simulink model "AFC_ensemble_other"  (R2022a)
settings: Solver=ode15s  StartTime=0.0  StopTime=T  MaxStep=.01  RelTol=1e-3
InitFcn:
  | seed_PA = randi(20000);
  | seed_ES = randi(20000);
StartFcn:
  | seed_PA = randi(20000);
  | seed_ES = randi(20000);
undefined symbols (not defined in the file): actionTable, actionUB, AF_ref_normal, AF_ref_power, AF_sensor_tol, change_freq_ES, change_freq_PA, edge_mu_max, fault_time, fuel_inj_max, fuel_inj_min, fuel_inj_tol, isAvg, isPred, isTerminate, isVote, kappa_tol, MAF_sensor_tol, max_Engine_Speed, max_Pedal_Angle, min_Engine_Speed, min_Pedal_Angle, mu_tol_normal, power_threshold, pump_tol, rewardToIndex, rewardUB1, rewardUB2, rewardWeights, stateTable, steady_mu_max, tau_ww_tol, time_tol, tranTable
libraries: rllib x9, simulink x2, dspstat3 x1
Description:
  | Modeling Engine Timing Using Triggered Subsystems
  | 
  | This example presents a model of a four-cylinder spark ignition engine
  | and demonstrates Simulink(R) capabilities to model an internal combustion
  | engine from the throttle to the crankshaft output. We used well-defined
  | physical principles supplemented, where appropriate, with empirical
  | relationships that describe the systems dynamic behavior without
  | introducing unnecessary complexity.
settings Model: ExtModeTrigMode=oneshot  ExtModeArmWhenConnect=off  Creator=The MathWorks Inc.  LastModifiedBy=momentumlab
settings SolverCC: ZeroCrossControl=DisableAll  AlgebraicLoopSolver=TrustRegion
settings DataIOCC: ExternalInput=[t__, u__]  SaveFormat=StructureWithTime  DSMLogging=off  ReturnWorkspaceOutputs=off
settings OptimizationCC: BlockReduction=off  BooleanDataType=off  LifeSpan=inf
settings DebuggingCC: SaveWithParameterizedLinksMsg=none  UnderspecifiedInitializationDetection=Classic  MergeDetectMultiDrivingBlocksExec=none  SignalResolutionControl=TryResolveAllWithWarning  ParameterPrecisionLossMsg=none  UnconnectedInputMsg=warning  UnconnectedOutputMsg=warning  UnconnectedLineMsg=warning  SFUnexpectedBacktrackingDiag=warning  SFNoUnconditionalDefaultTransitionDiag=warning  SFExecutionAtInitializationDiag=none  SFMachineParentedDataDiag=warning  ArithmeticOperatorsInVariantConditions=warning
settings HardwareCC: ProdBitPerPointer=32  ProdBitPerSizeT=32  ProdBitPerPtrDiffT=32  ProdLargestAtomicFloat=None  ProdIntDivRoundTo=Undefined  ProdEndianess=Unspecified  ProdWordSize=32  ProdHWDeviceType=32-bit Generic  TargetBitPerLong=64  TargetBitPerPointer=64  TargetBitPerSizeT=64  TargetBitPerPtrDiffT=64  TargetLongLongMode=on  TargetIntDivRoundTo=Zero  TargetEndianess=LittleEndian  TargetWordSize=64  TargetHWDeviceType=MATLAB Host  ProdEqTarget=off
settings ModelReferenceCC: PropagateSignalLabelsOutOfModel=off
settings SFSimCC: SimUseLocalCustomCode=off  CustomCodeUndefinedFunction=UseInterfaceOnly
settings RTWCC: RTWUseLocalCustomCode=off  DLArmComputeVersion=19.05
settings CodeAppCC: StateflowObjectComments=on
settings GRTTargetCC: TargetLangStandard=C89/C90 (ANSI)
settings ConfigComp: CovMetricSettings=d  CovSaveCumulativeToWorkspaceVar=on  CovSaveSingleToWorkspaceVar=on  CovExternalEMLEnable=off

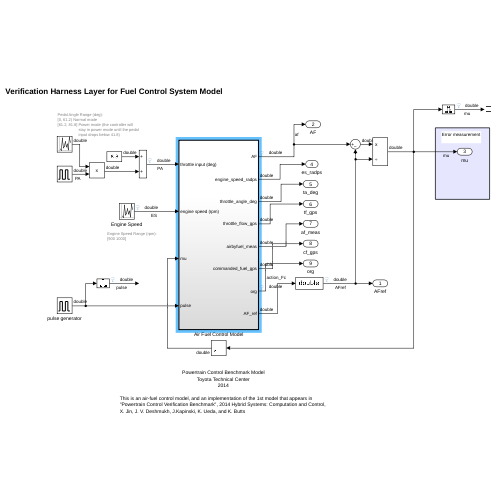
[thumbnail: Simulink's stored preview of the top-level diagram]
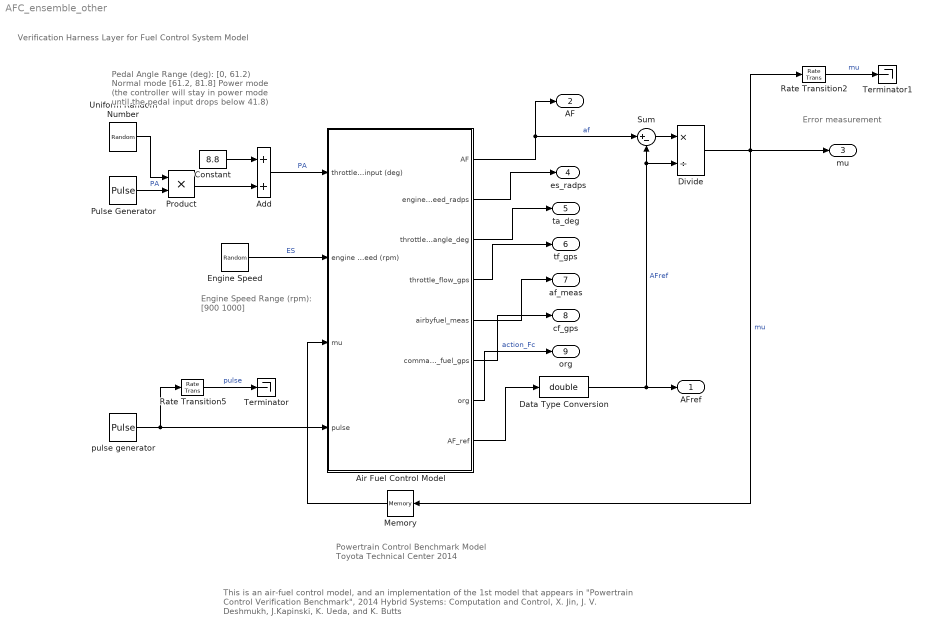
== system AFC_ensemble_other ==
  note: Error measurement
  note: Pedal Angle Range (deg):
      | [0, 61.2) Normal mode
      | [61.2, 81.8] Power mode (the controller will
      |                    stay in power mode until the pedal
      |                    input drops below 41.8)
  note: This is an air-fuel control model, and an implementation of the 1st model that appears in
      | "Powertrain Control Verification Benchmark", 2014 Hybrid Systems: Computation and Control,
      | X. Jin, J. V. Deshmukh, J.Kapinski, K. Ueda, and K. Butts
  note: Engine Speed Range (rpm):
      | [900 1000]
  note: Powertrain Control Benchmark Model
      | Toyota Technical Center
      | 2014
  note: Verification Harness Layer for Fuel Control System Model
  Add : Sum
  Air Fuel Control Model : Subsystem  Priority=1  TreatAsAtomicUnit=on
  Constant : Constant  Value=8.8
  Data Type Conversion : DataTypeConversion  OutDataTypeStr=double  SaturateOnIntegerOverflow=off  RndMeth=Floor
  Divide : Product  Inputs=*/
  Engine Speed : UniformRandomNumber  Minimum=min_Engine_Speed  Maximum=max_Engine_Speed  Seed=seed_ES  SampleTime=change_freq_ES  VectorParams1D=off
  Memory : Memory
  Product : Product
  Pulse Generator : DiscretePulseGenerator  PulseType=Time based  Period=change_freq_PA  PulseWidth=50
  Rate Transition2 : RateTransition  OutPortSampleTime=Ts_sample
  Rate Transition5 : RateTransition  OutPortSampleTime=Ts_sample
  Sum : Sum  Inputs=|+-
  Terminator : Terminator
  Terminator1 : Terminator
  Uniform Random Number : UniformRandomNumber  Minimum=min_Pedal_Angle  Maximum=max_Pedal_Angle  Seed=seed_PA  SampleTime=change_freq_PA
  pulse generator : DiscretePulseGenerator  PulseType=Time based  Period=change_freq_ES  PulseWidth=50  PhaseDelay=0.3
  AFref : Outport  VectorParamsAs1DForOutWhenUnconnected=off
  AF : Outport  Port=2  VectorParamsAs1DForOutWhenUnconnected=off
  mu : Outport  Port=3  VectorParamsAs1DForOutWhenUnconnected=off
  es_radps : Outport  Port=4
  ta_deg : Outport  Port=5
  tf_gps : Outport  Port=6
  af_meas : Outport  Port=7
  cf_gps : Outport  Port=8
  org : Outport  Port=9
  wires:
  Air Fuel Control Model/1(AF) -> AF/1, Sum/1  "af"
  Add/1 -> Air Fuel Control Model/1(throttle input (deg))  "PA"
  Air Fuel Control Model/8(AF_ref) -> Data Type Conversion/1
  Engine Speed/1 -> Air Fuel Control Model/2(engine speed (rpm))  "ES"
  Data Type Conversion/1 -> Sum/2, Divide/2, AFref/1  "AFref"
  Sum/1 -> Divide/1
  Air Fuel Control Model/2(engine_speed_radps) -> es_radps/1
  Air Fuel Control Model/3(throttle_angle_deg) -> ta_deg/1
  Air Fuel Control Model/4(throttle_flow_gps) -> tf_gps/1
  Air Fuel Control Model/5(airbyfuel_meas) -> af_meas/1
  Air Fuel Control Model/6(commanded_fuel_gps) -> cf_gps/1
  Air Fuel Control Model/7(org) -> org/1  "action_Fc"
  Divide/1 -> mu/1, Memory/1, Rate Transition2/1  "mu"
  Memory/1 -> Air Fuel Control Model/3(mu)
  Pulse Generator/1 -> Product/2  "PA"
  Uniform Random Number/1 -> Product/1
  Constant/1 -> Add/1
  Product/1 -> Add/2
  pulse generator/1 -> Rate Transition5/1, Air Fuel Control Model/4(pulse)
  Rate Transition5/1 -> Terminator/1  "pulse"
  Rate Transition2/1 -> Terminator1/1  "mu"

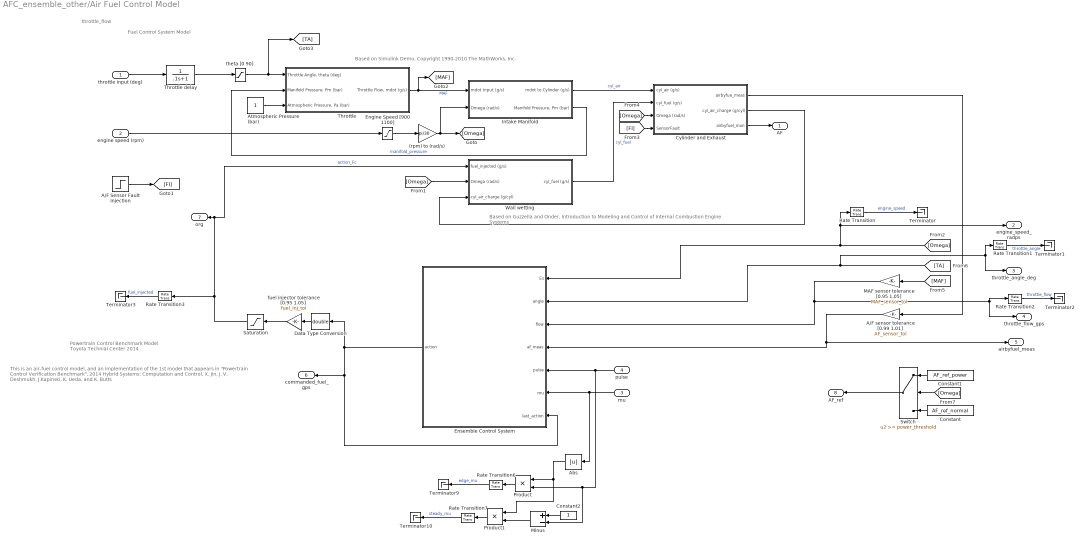
== system AFC_ensemble_other/Air Fuel Control Model ==
  note: throttle_flow
  note: Based on Simulink Demo, Copyright 1990-2010 The MathWorks, Inc.
  note: Based on Guzzella and Onder, Introduction to Modeling and Control of Internal Combustion Engine Systems
  note: Fuel Control System Model
  note: This is an air-fuel control model, and an implementation of the 1st model that appears in
      | "Powertrain Control Verification Benchmark", 2014 Hybrid Systems: Computation and Control,
      | X. Jin, J. V. Deshmukh, J.Kapinski, K. Ueda, and K. Butts
  note: Powertrain Control Benchmark Model
      | Toyota Technial Center
      | 2014
  throttle input (deg) : Inport  Description=[0, 81.2]
      settings: AttributesFormatString=%<Description>
  engine speed (rpm) : Inport  Description=[900,1100]  Port=2
      settings: AttributesFormatString=%<Description>
  mu : Inport  Port=3
  pulse : Inport  Port=4
  (rpm) to (rad/s) : Gain  Gain=pi/30
  A/F Sensor Fault Injection : Step  Time=fault_time  SampleTime=0
      settings: AttributesFormatString=1: Failure\n0: Normal
  A/F sensor tolerance [0.99 1.01] : Gain  Gain=AF_sensor_tol
  Abs : Abs  SaturateOnIntegerOverflow=off
  Atmospheric Pressure (bar) : Constant
  Constant : Constant  Value=AF_ref_normal
  Constant1 : Constant  Value=AF_ref_power
  Constant2 : Constant
  Cylinder and Exhaust : Subsystem
  Data Type Conversion : DataTypeConversion  OutDataTypeStr=double  SaturateOnIntegerOverflow=off  RndMeth=Floor
  Engine Speed [900 1100] : Saturate  UpperLimit=1100  LowerLimit=900
  Ensemble Control System : Subsystem
  Intake Manifold : Subsystem
  MAF sensor tolerance [0.95 1.05] : Gain  Gain=MAF_sensor_tol
  Minus : Sum  Inputs=+-
  Product : Product
  Product1 : Product
  Rate Transition{,1..3,6..7} (6 alike) : RateTransition  OutPortSampleTime=Ts_sample
  Saturation : Saturate  UpperLimit=fuel_inj_max  LowerLimit=fuel_inj_min
  Switch : Switch  Threshold=power_threshold  SaturateOnIntegerOverflow=off  InputSameDT=off
  Terminator{,1..3,9..10} (6 alike) : Terminator
  Throttle : Subsystem
  Throttle delay : TransferFcn  Denominator=[.1 1]
  Wall wetting : Subsystem
  fuel injector tolerance [0.95 1.05] : Gain  Gain=fuel_inj_tol
  theta [0 90] : Saturate  UpperLimit=90  LowerLimit=0
  AF : Outport  VectorParamsAs1DForOutWhenUnconnected=off
  engine_speed_radps : Outport  Port=2
  throttle_angle_deg : Outport  Port=3
  throttle_flow_gps : Outport  Port=4
  airbyfuel_meas : Outport  Port=5
  commanded_fuel_gps : Outport  Port=6
  org : Outport  Port=7
  AF_ref : Outport  Port=8
  wires:
  (rpm) to (rad/s)/1 -> [Omega], Intake Manifold/2(Omega (rad/s))
  Data Type Conversion/1 -> fuel injector tolerance [0.95 1.05]/1
  theta [0 90]/1 -> Throttle/1("Throttle Angle, theta (deg)"), [TA]
  Engine Speed [900 1100]/1 -> (rpm) to (rad/s)/1
  Cylinder and Exhaust/3("airbyfuel_mon ") -> AF/1
  MAF sensor tolerance [0.95 1.05]/1 -> Ensemble Control System/3(flow), throttle_flow_gps/1, Rate Transition2/1
  A/F sensor tolerance [0.99 1.01]/1 -> airbyfuel_meas/1, Ensemble Control System/4(af_meas)
  [MAF] -> MAF sensor tolerance [0.95 1.05]/1
  Cylinder and Exhaust/1(airbyfue_meas) -> A/F sensor tolerance [0.99 1.01]/1
  Throttle/1("Throttle Flow, mdot (g/s)") -> [MAF], Intake Manifold/1(mdot Input (g/s))  "MAF"
  Intake Manifold/2("Manifold Pressure, Pm (bar)") -> Throttle/2("Manifold Pressure, Pm (bar)")  "manifold_pressure"
  Atmospheric Pressure (bar)/1 -> Throttle/3("Atmospheric Pressure, Pa (bar) ")
  Wall wetting/1(cyl_fuel (g/s)) -> Cylinder and Exhaust/2(cyl_fuel (g/s))  "cyl_fuel"
  Intake Manifold/1(mdot to Cylinder (g/s)) -> Cylinder and Exhaust/1(cyl_air (g/s))  "cyl_air"
  [Omega] -> Cylinder and Exhaust/3(Omega (rad/s))
  [Omega] -> Wall wetting/2(Omega (rad/s))
  Cylinder and Exhaust/2(cyl_air_charge (g/cyl)) -> Wall wetting/3(cyl_air_charge (g/cyl))
  A/F Sensor Fault Injection/1 -> [FI]
  [FI] -> Cylinder and Exhaust/4(SensorFault)
  [TA] -> Ensemble Control System/2(angle), Rate Transition1/1, throttle_angle_deg/1
  throttle input (deg)/1 -> Throttle delay/1
  engine speed (rpm)/1 -> Engine Speed [900 1100]/1
  Throttle delay/1 -> theta [0 90]/1
  fuel injector tolerance [0.95 1.05]/1 -> Saturation/1
  Saturation/1 -> Rate Transition3/1, Wall wetting/1(fuel_injected (g/s)), org/1  "action_Fc"
  [Omega] -> Switch/2
  Constant1/1 -> Switch/1
  Constant/1 -> Switch/3
  Switch/1 -> AF_ref/1
  Rate Transition/1 -> Terminator/1  "engine_speed"
  [Omega] -> Ensemble Control System/1(Es), engine_speed_radps/1, Rate Transition/1
  Rate Transition1/1 -> Terminator1/1  "throttle_angle"
  Rate Transition2/1 -> Terminator2/1  "throttle_flow"
  Rate Transition3/1 -> Terminator3/1  "fuel_injected"
  Ensemble Control System/1(action) -> Data Type Conversion/1, Ensemble Control System/7(last_action), commanded_fuel_gps/1
  Rate Transition6/1 -> Terminator9/1  "edge_mu"
  Abs/1 -> Product1/1, Product/1
  Constant2/1 -> Minus/1
  pulse/1 -> Product/2, Minus/2, Ensemble Control System/5(pulse)
  Product1/1 -> Rate Transition7/1
  Product/1 -> Rate Transition6/1
  Rate Transition7/1 -> Terminator10/1  "steady_mu"
  mu/1 -> Abs/1, Ensemble Control System/6(mu)
  Minus/1 -> Product1/2

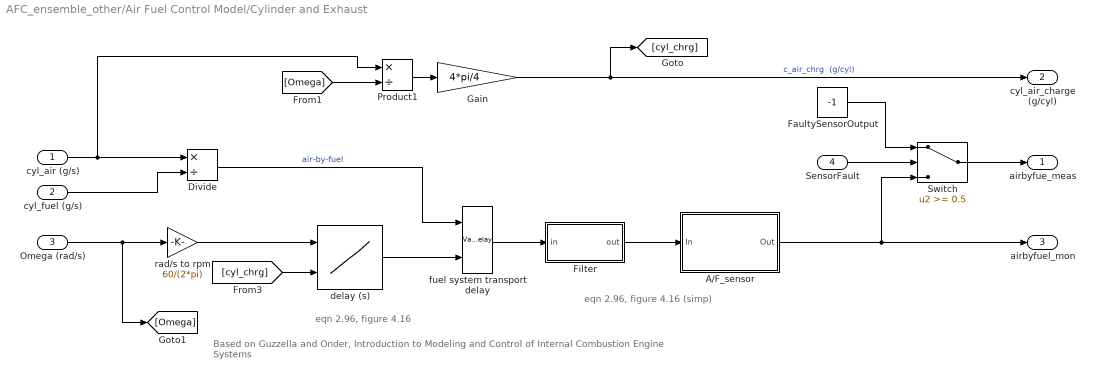
== system AFC_ensemble_other/Air Fuel Control Model/Cylinder and Exhaust ==
  note: Based on Guzzella and Onder, Introduction to Modeling and Control of Internal Combustion Engine Systems
  note: eqn 2.96, figure 4.16
  note: eqn 2.96, figure 4.16 (simp)
  cyl_air (g/s) : Inport
  cyl_fuel (g/s) : Inport  Port=2
  Omega (rad/s) : Inport  Port=3
  SensorFault : Inport  Port=4
  A/F_sensor : Subsystem
  Divide : Product  Inputs=*/
  FaultySensorOutput : Constant  Value=-1
  Filter : Subsystem
  Gain : Gain  Gain=4*pi/4
  Product1 : Product  Inputs=*/  RndMeth=Zero
  Switch : Switch  Threshold=0.5  SaturateOnIntegerOverflow=off  InputSameDT=off
  delay (s) : Lookup_n-D  BreakpointsForDimension1=[800,1000,1500,2000,3000]  BreakpointsForDimension2=[0.05,0.15,0.2,0.25]  Table=reshape([0.8,0.6,0.4,0.3,0.2,0.4,0.3,0.2,0.2,0.2,0.3,0.25,0.2,0.2,0.2,0.25,0.2,0.2,0.2,0.2],5,4)  UseLastTableValue=on  RndMeth=Simplest
      settings: InputPortMap=u0,u1
  fuel system transport delay : VariableTransportDelay  VariableDelayType=Variable transport delay  MaximumDelay=10  InitialOutput=14.7  MaximumPoints=20480
  rad/s to rpm : Gain  Gain=60/(2*pi)
  airbyfue_meas : Outport  VectorParamsAs1DForOutWhenUnconnected=off
  cyl_air_charge (g/cyl) : Outport  Port=2  VectorParamsAs1DForOutWhenUnconnected=off
  "airbyfuel_mon " : Outport  Port=3  VectorParamsAs1DForOutWhenUnconnected=off
  wires:
  cyl_air (g/s)/1 -> Divide/1, Product1/1
  [Omega] -> Product1/2
  Product1/1 -> Gain/1
  Gain/1 -> [cyl_chrg], cyl_air_charge (g/cyl)/1  "c_air_chrg  (g/cyl)"
  [cyl_chrg] -> delay (s)/2
  cyl_fuel (g/s)/1 -> Divide/2
  Omega (rad/s)/1 -> [Omega], rad/s to rpm/1
  rad/s to rpm/1 -> delay (s)/1
  delay (s)/1 -> fuel system transport delay/2
  fuel system transport delay/1 -> Filter/1(in)
  Switch/1 -> airbyfue_meas/1
  Divide/1 -> fuel system transport delay/1  "air-by-fuel"
  Filter/1(out) -> A/F_sensor/1(In)
  FaultySensorOutput/1 -> Switch/1
  SensorFault/1 -> Switch/2
  A/F_sensor/1(Out) -> Switch/3, "airbyfuel_mon "/1

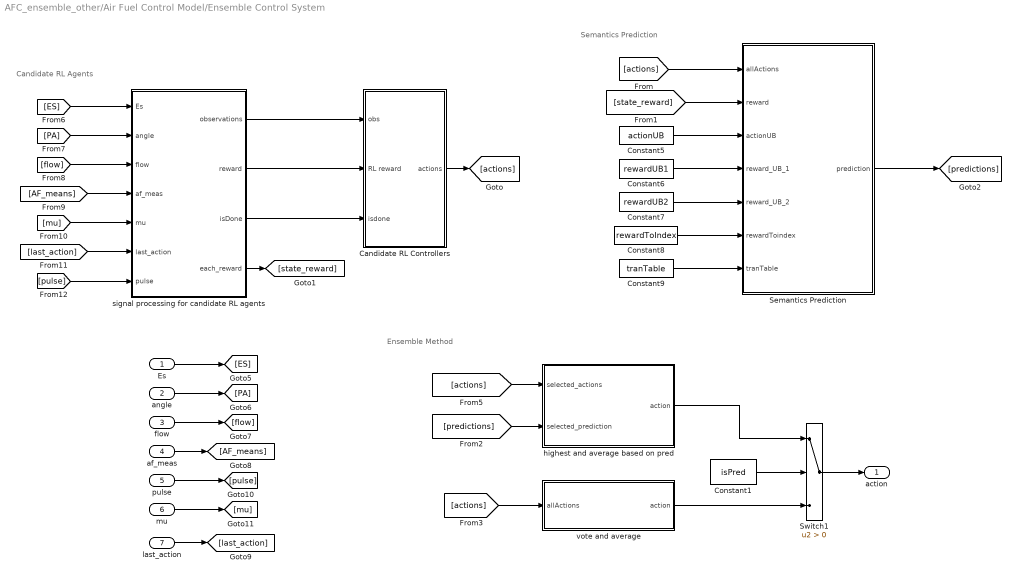
== system AFC_ensemble_other/Air Fuel Control Model/Ensemble Control System ==
  note: Candidate RL Agents
  note: Semantics Prediction
  note: Ensemble Method
  Es : Inport
  angle : Inport  Port=2
  flow : Inport  Port=3
  af_meas : Inport  Port=4
  pulse : Inport  Port=5
  mu : Inport  Port=6
  last_action : Inport  Port=7
  Candidate RL Controllers : Subsystem
  Constant1 : Constant  Value=isPred
  Constant5 : Constant  Value=actionUB
  Constant6 : Constant  Value=rewardUB1
  Constant7 : Constant  Value=rewardUB2
  Constant8 : Constant  Value=rewardToIndex
  Constant9 : Constant  Value=tranTable
  Semantics Prediction : Subsystem
  Switch1 : Switch  Criteria=u2 > Threshold  SaturateOnIntegerOverflow=off  InputSameDT=off
  highest and average based on pred : Subsystem
  signal processing for candidate RL agents : Subsystem
  vote and average : Subsystem
  action : Outport
  wires:
  last_action/1 -> [last_action]
  signal processing for candidate RL agents/3(isDone) -> Candidate RL Controllers/3(isdone)
  Constant8/1 -> Semantics Prediction/6(rewardToindex)
  Candidate RL Controllers/1(actions) -> [actions]
  Semantics Prediction/1(prediction) -> [predictions]
  signal processing for candidate RL agents/4(each_reward) -> [state_reward]
  [state_reward] -> Semantics Prediction/2(reward)
  Constant9/1 -> Semantics Prediction/7(tranTable)
  Constant5/1 -> Semantics Prediction/3(actionUB)
  Constant6/1 -> Semantics Prediction/4(reward_UB_1)
  [actions] -> Semantics Prediction/1(allActions)
  Constant7/1 -> Semantics Prediction/5(reward_UB_2)
  signal processing for candidate RL agents/2(reward) -> Candidate RL Controllers/2(RL reward)
  signal processing for candidate RL agents/1(observations) -> Candidate RL Controllers/1(obs)
  Es/1 -> [ES]
  angle/1 -> [PA]
  flow/1 -> [flow]
  af_meas/1 -> [AF_means]
  pulse/1 -> [pulse]
  mu/1 -> [mu]
  [ES] -> signal processing for candidate RL agents/1(Es)
  [PA] -> signal processing for candidate RL agents/2(angle)
  [flow] -> signal processing for candidate RL agents/3(flow)
  [AF_means] -> signal processing for candidate RL agents/4(af_meas)
  [mu] -> signal processing for candidate RL agents/5(mu)
  [last_action] -> signal processing for candidate RL agents/6(last_action)
  [pulse] -> signal processing for candidate RL agents/7(pulse)
  Constant1/1 -> Switch1/2
  [actions] -> vote and average/1(allActions)
  vote and average/1(action) -> Switch1/3
  highest and average based on pred/1(action) -> Switch1/1
  Switch1/1 -> action/1
  [predictions] -> highest and average based on pred/2(selected_prediction)
  [actions] -> highest and average based on pred/1(selected_actions)

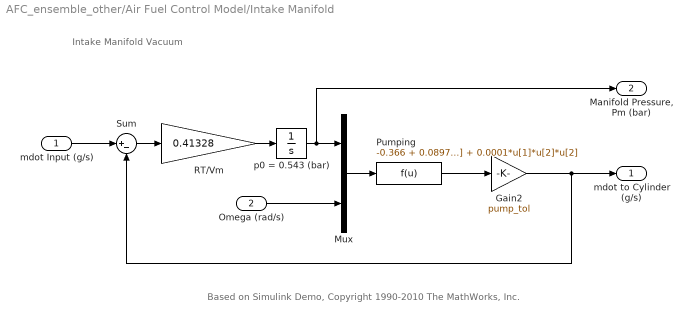
== system AFC_ensemble_other/Air Fuel Control Model/Intake Manifold ==
  note: Intake Manifold Vacuum
  note: Based on Simulink Demo, Copyright 1990-2010 The MathWorks, Inc.
  mdot Input (g/s) : Inport
  Omega (rad/s) : Inport  Port=2
  Gain2 : Gain  Gain=pump_tol  ParamDataTypeStr=single  OutDataTypeStr=Inherit: Inherit via back propagation  RndMeth=Simplest  SaturateOnIntegerOverflow=on
      settings: AttributesFormatString=pumping tolerance [0.9 1.1]
  Mux : Mux  Inputs=2
  Pumping : Fcn  Expr=-0.366 + 0.08979*u[1]*u[2] - 0.0337*u[2]*u[1]*u[1] + 0.0001*u[1]*u[2]*u[2]
  RT/Vm : Gain  Gain=0.41328  SaturateOnIntegerOverflow=on  OutDataTypeStr=Inherit: Same as input  ParamDataTypeStr=Inherit: Same as input
  Sum : Sum  Inputs=|+-  InputSameDT=on  SaturateOnIntegerOverflow=on  OutDataTypeStr=Inherit: Same as first input
  p0 = 0.543 (bar) : Integrator  InitialCondition=0.982
  mdot to Cylinder (g/s) : Outport  InitialOutput=0  VectorParamsAs1DForOutWhenUnconnected=off
  "Manifold Pressure, Pm (bar)" : Outport  Port=2  InitialOutput=0  VectorParamsAs1DForOutWhenUnconnected=off
  wires:
  mdot Input (g/s)/1 -> Sum/1
  RT/Vm/1 -> p0 = 0.543 (bar)/1
  Omega (rad/s)/1 -> Mux/2
  Mux/1 -> Pumping/1
  p0 = 0.543 (bar)/1 -> Mux/1, "Manifold Pressure, Pm (bar)"/1
  Sum/1 -> RT/Vm/1
  Pumping/1 -> Gain2/1
  Gain2/1 -> Sum/2, mdot to Cylinder (g/s)/1

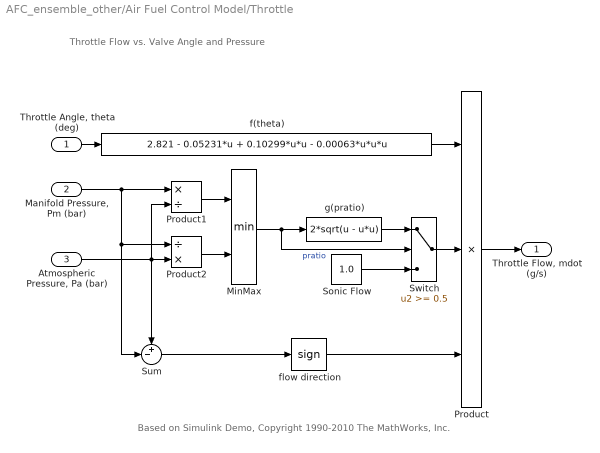
== system AFC_ensemble_other/Air Fuel Control Model/Throttle ==
  note: Throttle Flow vs. Valve Angle and Pressure
  note: Based on Simulink Demo, Copyright 1990-2010 The MathWorks, Inc.
  "Throttle Angle, theta (deg)" : Inport
  "Manifold Pressure, Pm (bar)" : Inport  Port=2
  "Atmospheric Pressure, Pa (bar) " : Inport  Port=3
  MinMax : MinMax  Inputs=2  InputSameDT=on  SaturateOnIntegerOverflow=on
  Product : Product  Inputs=3  InputSameDT=on  RndMeth=Zero  SaturateOnIntegerOverflow=on  OutDataTypeStr=Inherit: Same as first input
  Product1 : Product  Inputs=*/  InputSameDT=on  RndMeth=Zero  SaturateOnIntegerOverflow=on  OutDataTypeStr=Inherit: Same as first input
  Product2 : Product  Inputs=/*  InputSameDT=on  RndMeth=Zero  SaturateOnIntegerOverflow=on  OutDataTypeStr=Inherit: Same as first input
  "Sonic Flow " : Constant  Value=1.0
  Sum : Sum  Inputs=+-|  InputSameDT=on  SaturateOnIntegerOverflow=on  OutDataTypeStr=Inherit: Same as first input
  Switch : Switch  Threshold=0.5
  f(theta) : Fcn  Expr=2.821 - 0.05231*u + 0.10299*u*u - 0.00063*u*u*u
  flow direction : Signum
  g(pratio) : Fcn  Expr=2*sqrt(u - u*u)
  "Throttle Flow, mdot (g/s)" : Outport  InitialOutput=0  VectorParamsAs1DForOutWhenUnconnected=off
  wires:
  "Manifold Pressure, Pm (bar)"/1 -> Sum/2, Product2/1, Product1/1
  Product2/1 -> MinMax/2
  Product1/1 -> MinMax/1
  "Atmospheric Pressure, Pa (bar) "/1 -> Sum/1, Product2/2, Product1/2
  g(pratio)/1 -> Switch/1
  "Sonic Flow "/1 -> Switch/3
  Switch/1 -> Product/2
  flow direction/1 -> Product/3
  Sum/1 -> flow direction/1
  MinMax/1 -> g(pratio)/1, Switch/2  "pratio"
  "Throttle Angle, theta (deg)"/1 -> f(theta)/1
  Product/1 -> "Throttle Flow, mdot (g/s)"/1
  f(theta)/1 -> Product/1

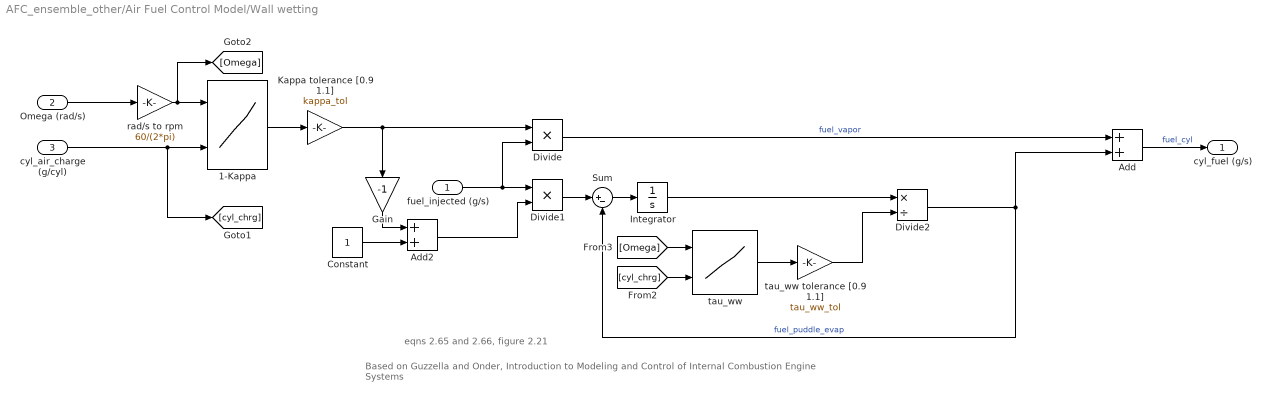
== system AFC_ensemble_other/Air Fuel Control Model/Wall wetting ==
  note: Based on Guzzella and Onder, Introduction to Modeling and Control of Internal Combustion Engine Systems
  note: eqns 2.65 and 2.66, figure 2.21
  fuel_injected (g/s) : Inport
  Omega (rad/s) : Inport  Port=2
  cyl_air_charge (g/cyl) : Inport  Port=3
  1-Kappa : Lookup_n-D  BreakpointsForDimension1=[1000,1500,2000,2500,3000]  BreakpointsForDimension2=[.1,.2,.3,.4]  Table=reshape([0.8,.7,.7,.8,.9,.7,.66,.65,.73,.85,.66,.66,.63,.66,.8,.6,.6,.6,.6,.7],5,4)  UseLastTableValue=on  RndMeth=Simplest
      settings: InputPortMap=u0,u1
  Add : Sum
  Add2 : Sum
  Constant : Constant
  Divide : Product  Inputs=**
  Divide1 : Product  Inputs=**
  Divide2 : Product  Inputs=*/
  Gain : Gain  Gain=-1
  Integrator : Integrator  InitialCondition=.0112
  Kappa tolerance [0.9 1.1] : Gain  Gain=kappa_tol
  Sum : Sum  Inputs=|+-
  rad/s to rpm : Gain  Gain=60/(2*pi)
  tau_ww : Lookup_n-D  BreakpointsForDimension1=[1000,1500,2000,2500,3000]  BreakpointsForDimension2=[0.1,0.2,0.3,0.4]  Table=reshape([.4,.3,.35,.3,.2,.22,.22,.4,.35,.5,.20,.22,.5,.4,.35,.35,.3,.45,.5,.4],5,4)  UseLastTableValue=on  RndMeth=Simplest
      settings: InputPortMap=u0,u1
  tau_ww tolerance [0.9 1.1] : Gain  Gain=tau_ww_tol
  cyl_fuel (g/s) : Outport  VectorParamsAs1DForOutWhenUnconnected=off
  wires:
  1-Kappa/1 -> Kappa tolerance [0.9 1.1]/1
  fuel_injected (g/s)/1 -> Divide/2, Divide1/1
  Divide/1 -> Add/1  "fuel_vapor"
  Add/1 -> cyl_fuel (g/s)/1  "fuel_cyl"
  Integrator/1 -> Divide2/1
  Divide1/1 -> Sum/1
  Sum/1 -> Integrator/1
  Divide2/1 -> Add/2, Sum/2  "fuel_puddle_evap"
  Add2/1 -> Divide1/2
  cyl_air_charge (g/cyl)/1 -> 1-Kappa/2, [cyl_chrg]
  [cyl_chrg] -> tau_ww/2
  tau_ww/1 -> tau_ww tolerance [0.9 1.1]/1
  Gain/1 -> Add2/1
  Constant/1 -> Add2/2
  rad/s to rpm/1 -> [Omega], 1-Kappa/1
  Omega (rad/s)/1 -> rad/s to rpm/1
  Kappa tolerance [0.9 1.1]/1 -> Divide/1, Gain/1
  tau_ww tolerance [0.9 1.1]/1 -> Divide2/2
  [Omega] -> tau_ww/1

== system AFC_ensemble_other/Air Fuel Control Model/Cylinder and Exhaust/A//F_sensor ==
  In : Inport
  A/F_sensor : Gain  OutDataTypeStr=double
  Filter : Subsystem
  Out : Outport  VectorParamsAs1DForOutWhenUnconnected=off
  wires:
  A/F_sensor/1 -> Out/1
  In/1 -> Filter/1(In)
  Filter/1(Out) -> A/F_sensor/1

== system AFC_ensemble_other/Air Fuel Control Model/Cylinder and Exhaust/Filter ==
  in : Inport
  Gain1 : Gain  Gain=10
  Integrator : Integrator  InitialCondition=14.7
  Sum : Sum  Inputs=|+-
  out : Outport  VectorParamsAs1DForOutWhenUnconnected=off
  wires:
  Integrator/1 -> out/1, Sum/2
  in/1 -> Sum/1
  Gain1/1 -> Integrator/1
  Sum/1 -> Gain1/1

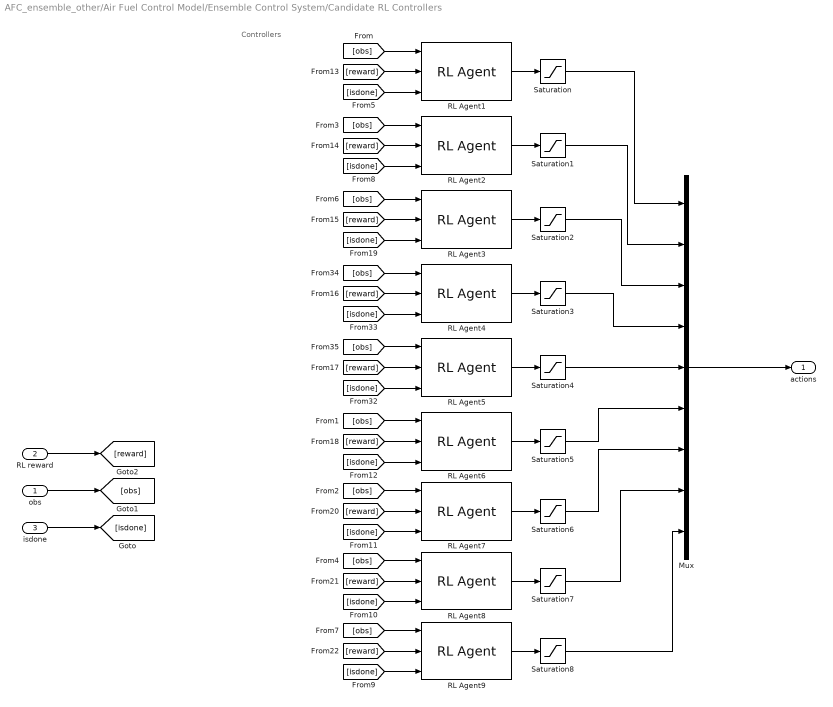
== system AFC_ensemble_other/Air Fuel Control Model/Ensemble Control System/Candidate RL Controllers ==
  note: Controllers
  obs : Inport
  RL reward : Inport  Port=2
  isdone : Inport  Port=3
  Mux : Mux  Inputs=9
  RL Agent1 : rllib/RL Agent  Agent=agent1  ExternalActionAsInput=off  ProvideLastAction=off  ProvideCumRwd=off  TreatAsDirectFeedthrough=on  UseStrictObservationDataTypes=off
  RL Agent2 : rllib/RL Agent  Agent=agent2  ExternalActionAsInput=off  ProvideLastAction=off  ProvideCumRwd=off  TreatAsDirectFeedthrough=on  UseStrictObservationDataTypes=off
  RL Agent3 : rllib/RL Agent  Agent=agent3  ExternalActionAsInput=off  ProvideLastAction=off  ProvideCumRwd=off  TreatAsDirectFeedthrough=on  UseStrictObservationDataTypes=off
  RL Agent4 : rllib/RL Agent  Agent=agent3  ExternalActionAsInput=off  ProvideLastAction=off  ProvideCumRwd=off  TreatAsDirectFeedthrough=on  UseStrictObservationDataTypes=off
  RL Agent5 : rllib/RL Agent  Agent=agent3  ExternalActionAsInput=off  ProvideLastAction=off  ProvideCumRwd=off  TreatAsDirectFeedthrough=on  UseStrictObservationDataTypes=off
  RL Agent6 : rllib/RL Agent  Agent=agent6  ExternalActionAsInput=off  ProvideLastAction=off  ProvideCumRwd=off  TreatAsDirectFeedthrough=on  UseStrictObservationDataTypes=off
  RL Agent7 : rllib/RL Agent  Agent=agent7  ExternalActionAsInput=off  ProvideLastAction=off  ProvideCumRwd=off  TreatAsDirectFeedthrough=on  UseStrictObservationDataTypes=off
  RL Agent8 : rllib/RL Agent  Agent=agent8  ExternalActionAsInput=off  ProvideLastAction=off  ProvideCumRwd=off  TreatAsDirectFeedthrough=on  UseStrictObservationDataTypes=off
  RL Agent9 : rllib/RL Agent  Agent=agent9  ExternalActionAsInput=off  ProvideLastAction=off  ProvideCumRwd=off  TreatAsDirectFeedthrough=on  UseStrictObservationDataTypes=off
  Saturation{,1..8} (9 alike) : Saturate  UpperLimit=fuel_inj_max  LowerLimit=fuel_inj_min
  actions : Outport
  wires:
  [obs] -> RL Agent7/1
  [obs] -> RL Agent4/1
  [obs] -> RL Agent3/1
  Saturation3/1 -> Mux/4
  [obs] -> RL Agent1/1
  [isdone] -> RL Agent1/3
  [obs] -> RL Agent2/1
  [obs] -> RL Agent5/1
  RL Agent1/1 -> Saturation/1
  [isdone] -> RL Agent8/3
  [isdone] -> RL Agent6/3
  Saturation/1 -> Mux/1
  RL Agent6/1 -> Saturation5/1
  Saturation4/1 -> Mux/5
  RL Agent3/1 -> Saturation2/1
  [isdone] -> RL Agent2/3
  [isdone] -> RL Agent7/3
  RL Agent8/1 -> Saturation7/1
  Saturation1/1 -> Mux/2
  [isdone] -> RL Agent5/3
  Mux/1 -> actions/1
  [obs] -> RL Agent6/1
  [isdone] -> RL Agent3/3
  RL Agent5/1 -> Saturation4/1
  RL Agent4/1 -> Saturation3/1
  RL Agent7/1 -> Saturation6/1
  RL Agent2/1 -> Saturation1/1
  [obs] -> RL Agent8/1
  Saturation2/1 -> Mux/3
  [isdone] -> RL Agent4/3
  RL Agent9/1 -> Saturation8/1
  [obs] -> RL Agent9/1
  [isdone] -> RL Agent9/3
  Saturation5/1 -> Mux/6
  Saturation6/1 -> Mux/7
  Saturation7/1 -> Mux/8
  Saturation8/1 -> Mux/9
  isdone/1 -> [isdone]
  obs/1 -> [obs]
  RL reward/1 -> [reward]
  [reward] -> RL Agent1/2
  [reward] -> RL Agent2/2
  [reward] -> RL Agent3/2
  [reward] -> RL Agent4/2
  [reward] -> RL Agent5/2
  [reward] -> RL Agent6/2
  [reward] -> RL Agent7/2
  [reward] -> RL Agent8/2
  [reward] -> RL Agent9/2

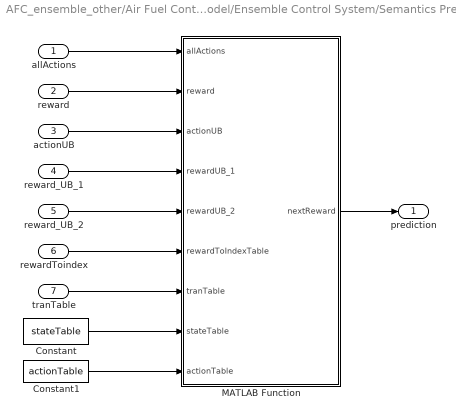
== system AFC_ensemble_other/Air Fuel Control Model/Ensemble Control System/Semantics Prediction ==
  allActions : Inport
  reward : Inport  Port=2
  actionUB : Inport  Port=3
  reward_UB_1 : Inport  Port=4
  reward_UB_2 : Inport  Port=5
  rewardToindex : Inport  Port=6
  tranTable : Inport  Port=7
  Constant : Constant  Value=stateTable
  Constant1 : Constant  Value=actionTable
  MATLAB Function : MATLAB Function  TreatAsAtomicUnit=on
  prediction : Outport
  wires:
  MATLAB Function/1(nextReward) -> prediction/1
  allActions/1 -> MATLAB Function/1(allActions)
  reward/1 -> MATLAB Function/2(reward)
  actionUB/1 -> MATLAB Function/3(actionUB)
  reward_UB_1/1 -> MATLAB Function/4(rewardUB_1)
  reward_UB_2/1 -> MATLAB Function/5(rewardUB_2)
  rewardToindex/1 -> MATLAB Function/6(rewardToIndexTable)
  tranTable/1 -> MATLAB Function/7(tranTable)
  Constant/1 -> MATLAB Function/8(stateTable)
  Constant1/1 -> MATLAB Function/9(actionTable)

== system AFC_ensemble_other/Air Fuel Control Model/Ensemble Control System/highest and average based on pred ==
  note: action with highest predicted reward
  note: average action based on predictions
  selected_actions : Inport
  selected_prediction : Inport  Port=2
  Constant : Constant  Value=isAvg
  Switch : Switch  Criteria=u2 > Threshold  SaturateOnIntegerOverflow=off  InputSameDT=off
  averaged action : MATLAB Function  TreatAsAtomicUnit=on
  one action : MATLAB Function  TreatAsAtomicUnit=on
  action : Outport
  wires:
  selected_actions/1 -> averaged action/1(allActions), one action/1(allActions)
  selected_prediction/1 -> one action/2(predications), averaged action/2(predications)
  one action/1(finalAction) -> Switch/3
  Switch/1 -> action/1
  Constant/1 -> Switch/2
  averaged action/1(finalAction) -> Switch/1

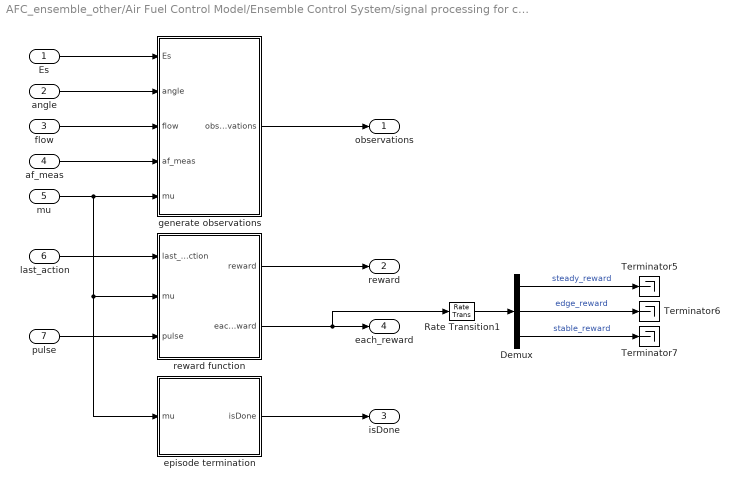
== system AFC_ensemble_other/Air Fuel Control Model/Ensemble Control System/signal processing for candidate RL agents ==
  Es : Inport
  angle : Inport  Port=2
  flow : Inport  Port=3
  af_meas : Inport  Port=4
  mu : Inport  Port=5
  last_action : Inport  Port=6
  pulse : Inport  Port=7
  Demux : Demux  Outputs=3
  Rate Transition1 : RateTransition  OutPortSampleTime=Ts_sample
  Terminator5 : Terminator
  Terminator6 : Terminator
  Terminator7 : Terminator
  episode termination : Subsystem
  generate observations : Subsystem
  reward function : Subsystem
  observations : Outport
  reward : Outport  Port=2
  isDone : Outport  Port=3
  each_reward : Outport  Port=4
  wires:
  angle/1 -> generate observations/2(angle)
  af_meas/1 -> generate observations/4(af_meas)
  mu/1 -> episode termination/1(mu), reward function/2(mu), generate observations/5(mu)
  reward function/2(each_reward) -> Rate Transition1/1, each_reward/1
  Es/1 -> generate observations/1(Es)
  reward function/1(reward) -> reward/1
  last_action/1 -> reward function/1(last_action)
  flow/1 -> generate observations/3(flow)
  pulse/1 -> reward function/3(pulse)
  episode termination/1(isDone) -> isDone/1
  generate observations/1(observations) -> observations/1
  Demux/3 -> Terminator7/1  "stable_reward"
  Demux/1 -> Terminator5/1  "steady_reward"
  Demux/2 -> Terminator6/1  "edge_reward"
  Rate Transition1/1 -> Demux/1

== system AFC_ensemble_other/Air Fuel Control Model/Ensemble Control System/vote and average ==
  note: Majority Vote
  note: Average
  allActions : Inport
  Constant : Constant  Value=actionUB
  Constant1 : Constant  Value=isVote
  Mean : dspstat3/Mean  run=off  InputProcessing=Columns as channels (frame based)  reset_popup=None  directionMode=Entire input  dimension=1  roiEnable=off  roiType=Rectangles  roiPortion=Entire ROI  roiOutput=Individual statistics for each ROI  roiFlag=off  roundingMode=Floor  overflowMode=off  outputDataTypeStr=Inherit: Same as accumulator  outputMin=[]  outputMax=[]  outputLastDataTypeStr=Inherit: Same as accumulator
  Switch : Switch  Criteria=u2 > Threshold  SaturateOnIntegerOverflow=off  InputSameDT=off
  majority voting : MATLAB Function  TreatAsAtomicUnit=on
  action : Outport
  wires:
  allActions/1 -> Mean/1, majority voting/1(allActions)
  Switch/1 -> action/1
  Constant/1 -> majority voting/2(actionUB)
  majority voting/1(actionOut) -> Switch/1
  Mean/1 -> Switch/3
  Constant1/1 -> Switch/2

== system AFC_ensemble_other/Air Fuel Control Model/Cylinder and Exhaust/A//F_sensor/Filter ==
  In : Inport
  Gain : Gain  Gain=50
  Integrator : Integrator  InitialCondition=14.7
  Sum : Sum  Inputs=|+-
  Out : Outport  VectorParamsAs1DForOutWhenUnconnected=off
  wires:
  Integrator/1 -> Out/1, Sum/2
  In/1 -> Sum/1
  Gain/1 -> Integrator/1
  Sum/1 -> Gain/1

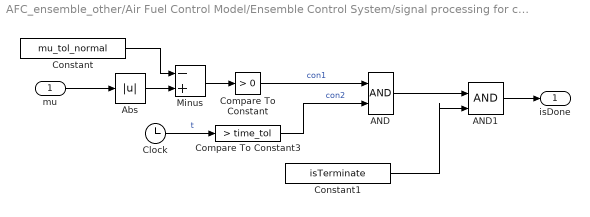
== system AFC_ensemble_other/Air Fuel Control Model/Ensemble Control System/signal processing for candidate RL agents/episode termination ==
  mu : Inport
  AND : Logic  IconShape=distinctive  AllPortsSameDT=off  OutDataTypeStr=boolean
  AND1 : Logic  IconShape=distinctive  AllPortsSameDT=off  OutDataTypeStr=boolean
  Abs : Abs  SaturateOnIntegerOverflow=off
  Clock : Clock
  Compare To Constant : simulink/Logic and Bit Operations/Compare To Constant  relop=>  const=0  OutDataTypeStr=boolean
  Compare To Constant3 : simulink/Logic and Bit Operations/Compare To Constant  relop=>  const=time_tol  OutDataTypeStr=boolean
  Constant : Constant  Value=mu_tol_normal
  Constant1 : Constant  Value=isTerminate
  Minus : Sum  Inputs=-+
  isDone : Outport
  wires:
  Compare To Constant/1 -> AND/1  "con1"
  Clock/1 -> Compare To Constant3/1  "t"
  Compare To Constant3/1 -> AND/2  "con2"
  AND/1 -> AND1/1
  Constant/1 -> Minus/1
  mu/1 -> Abs/1
  Minus/1 -> Compare To Constant/1
  Abs/1 -> Minus/2
  Constant1/1 -> AND1/2
  AND1/1 -> isDone/1

== system AFC_ensemble_other/Air Fuel Control Model/Ensemble Control System/signal processing for candidate RL agents/generate observations ==
  Es : Inport
  angle : Inport  Port=2
  flow : Inport  Port=3
  af_meas : Inport  Port=4
  mu : Inport  Port=5
  Mux : Mux  Inputs=5
  observations : Outport
  wires:
  Es/1 -> Mux/1
  Mux/1 -> observations/1
  af_meas/1 -> Mux/4
  angle/1 -> Mux/2
  flow/1 -> Mux/3
  mu/1 -> Mux/5

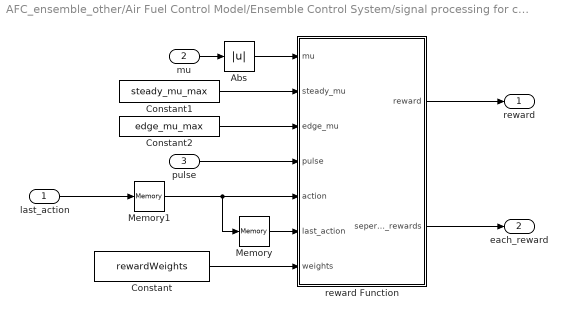
== system AFC_ensemble_other/Air Fuel Control Model/Ensemble Control System/signal processing for candidate RL agents/reward function ==
  last_action : Inport
  mu : Inport  Port=2
  pulse : Inport  Port=3
  Abs : Abs  SaturateOnIntegerOverflow=off
  Constant : Constant  Value=rewardWeights
  Constant1 : Constant  Value=steady_mu_max
  Constant2 : Constant  Value=edge_mu_max
  Memory : Memory  InheritSampleTime=on
  Memory1 : Memory  InheritSampleTime=on
  reward Function : MATLAB Function  TreatAsAtomicUnit=on
  reward : Outport
  each_reward : Outport  Port=2
  wires:
  last_action/1 -> Memory1/1
  mu/1 -> Abs/1
  reward Function/1(reward) -> reward/1
  Abs/1 -> reward Function/1(mu)
  Constant/1 -> reward Function/7(weights)
  pulse/1 -> reward Function/4(pulse)
  Constant1/1 -> reward Function/2(steady_mu)
  Constant2/1 -> reward Function/3(edge_mu)
  Memory/1 -> reward Function/6(last_action)
  reward Function/2(seperate_rewards) -> each_reward/1
  Memory1/1 -> reward Function/5(action), Memory/1

== matlab function AFC_ensemble_other/Air Fuel Control Model/Ensemble Control System/signal processing for candidate RL agents/reward function/reward Function ==
  data: mu input; reward output; steady_mu input; edge_mu input; pulse input; action input; last_action input; weights input; seperate_rewards output
function [reward,seperate_rewards] = reward_fun(mu, steady_mu, edge_mu, pulse, action, last_action, weights)
    
    % reward for steady-state
    steadyError = mu - steady_mu;
    if steadyError <= 0
        steadyReward = tanh(abs(steadyError)*150);
%         steadyReward = tanh(abs(steadyError)*30);

    else
        steadyReward = -tanh(steadyError*1.5);
%         steadyReward = -tanh(steadyError/1.5);
    end
    
    % reward for edge
    edgeError = mu - edge_mu;
    if edgeError <= 0
        edgeReward = tanh(abs(edgeError)*50);
    else
        edgeReward = -tanh(edgeError*1.5);
%         edgeReward = -tanh(edgeError/1.5);
    end
    
    % reward for stability
    stableError = -tanh(abs(action-last_action)*2);

    % final reward
    reward = weights(1)*steadyReward + weights(2)*edgeReward + weights(3)*stableError + 0.1;
%     reward = steadyReward + 0.1;
    seperate_rewards = [steadyReward, edgeReward,stableError];

== matlab function AFC_ensemble_other/Air Fuel Control Model/Ensemble Control System/Semantics Prediction/MATLAB Function ==
  data: allActions input; nextReward output; reward input; actionUB input; rewardUB_1 input; rewardUB_2 input; rewardToIndexTable input; tranTable input; stateTable input; actionTable input
function nextReward  = fcn(allActions, reward, actionUB, rewardUB_1,rewardUB_2, rewardToIndexTable, tranTable, stateTable,actionTable)

numController = 9;

nextReward = ones(numController, 1);
abReward_1 = find(rewardUB_1 >= reward(1), 1, 'first');  % concrete state -> abstract state
abReward_2 = find(rewardUB_2 >= reward(2), 1, 'first');

if isempty(abReward_1) || isempty(abReward_2)      % if this is an unseen reward
    nextReward = zeros(numController,1);
else
    rewardIndex1 = rewardToIndexTable(:,1)==abReward_1;
    rewardIndex2 = rewardToIndexTable(:,2)==abReward_2;
    
    if isempty(rewardIndex1) || isempty(rewardIndex2)      % if this is an unseen abstract state
        nextReward = zeros(numController,1);
    else
        abState = rewardToIndexTable(rewardToIndexTable(:,1)==abReward_1 & rewardToIndexTable(:,2)==abReward_2, 3);
        
        if isempty(abState)
            nextReward = zeros(numController,1);
        else
            for i = 1:numController
            
                action = allActions(i);
                abAction = find(actionUB >= action, 1, 'first');      % concrete action -> abstract action
            
                stateIndex = stateTable==abState;
                actionindex = actionTable==abAction;
            
                if isempty(stateIndex) || isempty(actionindex)  % if this is an unseen abstract state-action pair
                    abTranReward = 0;
                else
                    temp = stateIndex + actionindex;
                    if ismember(2,temp)
                        abTranReward = tranTable((stateIndex & actionindex),5);
                    else
                        abTranReward = 0;
                    end
                end
                nextReward(i,1) = abTranReward;
            end
        end
    end
end

== matlab function AFC_ensemble_other/Air Fuel Control Model/Ensemble Control System/vote and average/majority voting ==
  data: actionOut output; allActions input; actionUB input
function actionOut = fcn(allActions, actionUB)

numController = 9;

abstractAction = zeros(numController, 2);

for i = 1:numController
    abstractAction(i,1) = find(actionUB >= allActions(i), 1, 'first');      % concrete action -> abstract action;
    abstractAction(i,2) = allActions(i);
end

[GC,GR] = groupcounts(abstractAction(:,1));
actionIndex = GR(GC==max(GC));
actionIndex = ismember(abstractAction(:,1),actionIndex);
actionOut = mean(abstractAction(actionIndex,2));

== matlab function AFC_ensemble_other/Air Fuel Control Model/Ensemble Control System/highest and average based on pred/averaged action ==
  data: allActions input; finalAction output; predications input
function finalAction = fcn(allActions, predications)

% average of actions with top 3 highest predicted rewards

selectPred = predications(predications>=0);

if isempty(selectPred)
    actionPred = cat(2, allActions,predications);
    actionPred = sortrows(actionPred,2,'descend');
    finalAction = mean(actionPred(1:3,1));
else
    selectAction = allActions(predications>=0);
    actionPred = cat(2, selectAction,selectPred);
    actionPred = sortrows(actionPred,2,'descend');
    if length(actionPred) <3
        finalAction = mean(actionPred(:,1));
    else
        finalAction = mean(actionPred(1:3,1));
    end

end

== matlab function AFC_ensemble_other/Air Fuel Control Model/Ensemble Control System/highest and average based on pred/one action ==
  data: allActions input; finalAction output; predications input
function finalAction = fcn(allActions, predications)

% take the action with highest predicted reward
[~, idx] = max(predications);
finalAction = allActions(idx);
